simulink model "model1"  (R2024b)
settings: Solver=VariableStepAuto  StartTime=0.0  StopTime=10.0  MaxStep=1e-2  RelTol=1e-3
values from neighbouring files (symbols this model uses):
  A = [1,2;-3,-4]    [run1.m]    (also in run2.m; test.m = sqrt((Pival(1,1)*cos(alpha)+Pival(1,2)*cos(beta))^2+(Pival(1)
  Bw = 1    [design_extended.m]    (also in run1.m = [1;2]; run2.m = [2;1])
  C = [1,0;2,0;1,2]    [run1.m]    (also in run2.m = [1,0;1,0;1,1])
  Dw = [1;2]    [design_extended.m]    (also in run1.m = Cperp+C*[1;1]; run2.m = Cperp*1+0*C*[1;1]; test.m)
  Pival = proj(Dw)    [design_extended.m]    (also in run1.m = proj(C); run2.m = proj(C); test.m)
settings Model: Creator=Mehmet  LastModifiedBy=Mehmet

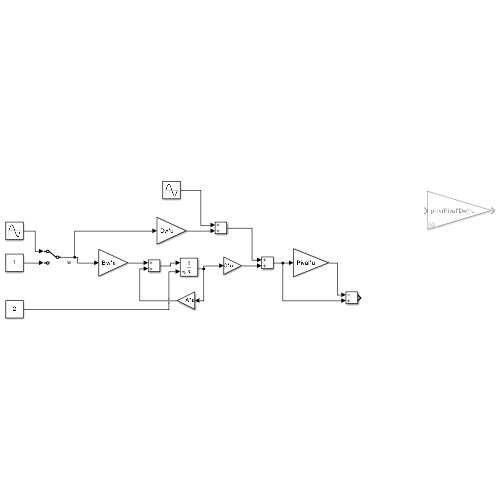
[thumbnail: Simulink's stored preview of the top-level diagram]
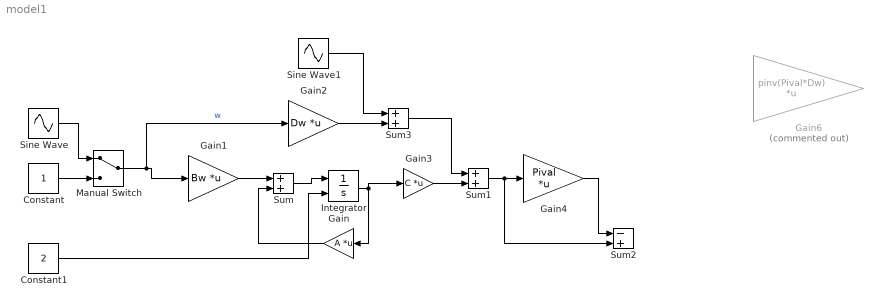
== system model1 ==
  Constant : Constant
  Constant1 : Constant  Value=2
  Gain : Gain  Gain=A  Multiplication=Matrix(K*u)
  Gain1 : Gain  Gain=Bw  Multiplication=Matrix(K*u)
  Gain2 : Gain  Gain=Dw  Multiplication=Matrix(K*u)
  Gain3 : Gain  Gain=C  Multiplication=Matrix(K*u)
  Gain4 : Gain  Gain=Pival  Multiplication=Matrix(K*u)
  Gain6 : Gain  Commented=on  Gain=pinv(Pival*Dw)  Multiplication=Matrix(K*u)
  Integrator : Integrator  InitialConditionSource=external
  Manual Switch : ManualSwitch
  Sine Wave : Sin  Frequency=5  SampleTime=0
  Sine Wave1 : Sin  Frequency=20  SampleTime=0
  Sum : Sum
  Sum1 : Sum
  Sum2 : Sum  Inputs=-+
  Sum3 : Sum
  wires:
  Gain/1 -> Sum/2
  Sum/1 -> Integrator/1
  Integrator/1 -> Gain3/1, Gain/1
  Gain1/1 -> Sum/1
  Gain3/1 -> Sum1/2
  Sum3/1 -> Sum1/1
  Sum1/1 -> Sum2/2, Gain4/1
  Gain4/1 -> Sum2/1
  Constant/1 -> Manual Switch/2
  Sine Wave/1 -> Manual Switch/1
  Manual Switch/1 -> Gain2/1, Gain1/1  "w"
  Constant1/1 -> Integrator/2
  Gain2/1 -> Sum3/2
  Sine Wave1/1 -> Sum3/1
